simulink model "experimento1_02_sim"  (R2014a)
settings: Solver=ode45  StartTime=0.0  StopTime=50  RelTol=1e-3
values from neighbouring files (symbols this model uses):
  A = [0 1 0; 0 0 1; -5.008 -25.1026 -5.0325]    [experimento1_01.m]
  B = [0; 25.04; -121.005]    [experimento1_01.m]
  C = [1 0 0]    [experimento1_01.m]
  D = 0    [experimento1_01.m]
settings Model: Creator=unieerisantos  LastModifiedBy=unieerisantos

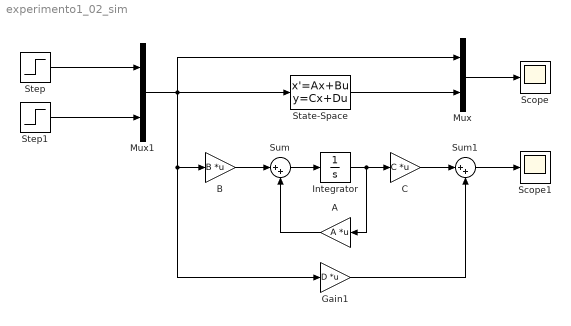
== system experimento1_02_sim ==
  A : Gain  Gain=A  Multiplication=Matrix(K*u)
  B : Gain  Gain=B  Multiplication=Matrix(K*u)
  C : Gain  Gain=C  Multiplication=Matrix(K*u)
  Gain1 : Gain  Gain=D  Multiplication=Matrix(K*u)
  Integrator : Integrator
  Mux : Mux  Inputs=2
  Mux1 : Mux  Inputs=2
  Scope : Scope
  Scope1 : Scope
  State-Space : StateSpace  A=A  B=B  C=C  D=D  X0=0
  Step : Step  Time=10  SampleTime=0
  Step1 : Step  Time=30  After=-1  SampleTime=0
  Sum : Sum  Inputs=|++
  Sum1 : Sum  Inputs=|++
  wires:
  Mux1/1 -> Gain1/1, B/1, State-Space/1, Mux/1
  Step/1 -> Mux1/1
  Step1/1 -> Mux1/2
  Mux/1 -> Scope/1
  B/1 -> Sum/1
  Sum/1 -> Integrator/1
  Integrator/1 -> A/1, C/1
  C/1 -> Sum1/1
  A/1 -> Sum/2
  Gain1/1 -> Sum1/2
  Sum1/1 -> Scope1/1
  State-Space/1 -> Mux/2
